simulink model "Simple_Model_Packaging_zhentouzhenwei3"  (R2022b)
settings: Solver=VariableStepAuto  StartTime=0.0  StopTime=0.05  RelTol=1e-3
InitFcn:
  | Parameter_Initialize_zhentouzhenwei
undefined symbols (not defined in the file or in its folder): gcbh, magnitude, model, rcfiltgaincompat
libraries: simulink x2, commrandsrc3 x2, commfilt2 x1, commchan3 x1, dspsigops x1, commdigbbndcpm2 x1, commseqgen3 x1, commutil2 x1, dsparch4 x1
settings Model: Creator=z0y  LastModifiedBy=z0y

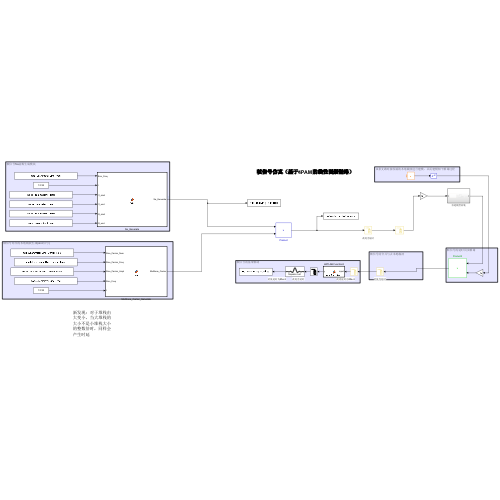
[thumbnail: Simulink's stored preview of the top-level diagram]
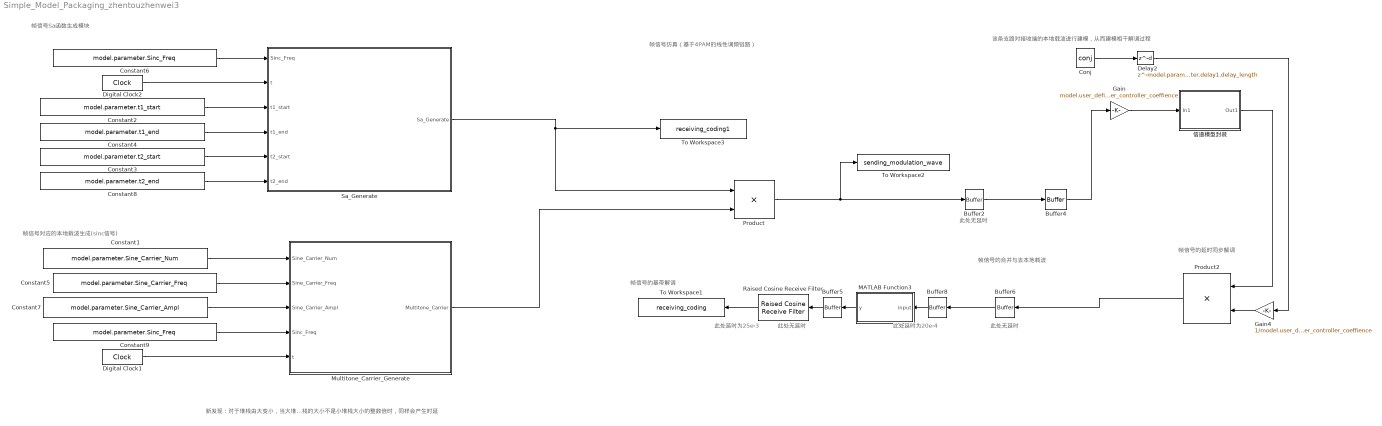
== system Simple_Model_Packaging_zhentouzhenwei3 ==
  note: 此处无延时
  note: 帧信号的延时同步解调
  note: 帧信号Sa函数生成模块
  note: 此处无延时
  note: 此处延时为25e-3
  note: 帧信号的基带解调
  note: 该条支路对接收端的本地载波进行建模，从而建模相干解调过程
  note: 帧信号的合并与去本地载波
  note: 帧信号仿真（基于4PAM的线性调频链路）
  note: 新发现：对于堆栈由大变小，当大堆栈的大小不是小堆栈大小的整数倍时，同样会产生时延
  note: 此处延时为20e-4
  note: 此处无延时
  note: 帧信号对应的本地载波生成(sinc信号)
  Buffer2 : Buffer  N=model.parameter.Buffer2.Output_buffer_size  OutputFrames=off
  Buffer4 : Buffer  N=model.parameter.Buffer4.Output_buffer_size  OutputFrames=off
  Buffer5 : Buffer  N=model.parameter.Buffer5.Output_buffer_size  OutputFrames=off
  Buffer6 : Buffer  N=model.parameter.Buffer6.Output_buffer_size  OutputFrames=off
  Buffer8 : Buffer  N=model.parameter.Buffer8.Output_buffer_size  OutputFrames=off
  Conj : Math  Operator=conj
  Constant1 : Constant  Value=model.parameter.Sine_Carrier_Num
  Constant2 : Constant  Value=model.parameter.t1_start
  Constant3 : Constant  Value=model.parameter.t2_start
  Constant4 : Constant  Value=model.parameter.t1_end
  Constant5 : Constant  Value=model.parameter.Sine_Carrier_Freq
  Constant6 : Constant  Value=model.parameter.Sinc_Freq
  Constant7 : Constant  Value=model.parameter.Sine_Carrier_Ampl
  Constant8 : Constant  Value=model.parameter.t2_end
  Constant9 : Constant  Value=model.parameter.Sinc_Freq
  Delay2 : Delay  DelayLength=model.parameter.delay1.delay_length  InitialCondition=0  InputProcessing=Columns as channels (frame based)
  Digital Clock1 : DigitalClock  SampleTime=model.parameter.Digital_Clock2.CarrierTs
  Digital Clock2 : DigitalClock  SampleTime=model.parameter.Digital_Clock2.CarrierTs
  Gain : Gain  Gain=model.user_defined.TR.Sig_power_controller_coeffience
  Gain4 : Gain  Gain=1/model.user_defined.TR.Sig_power_controller_coeffience
  MATLAB Function3 : MATLAB Function  TreatAsAtomicUnit=on
  Multitone_Carrier_Generate : MATLAB Function  TreatAsAtomicUnit=on
  Product : Product
  Product2 : Product
  Raised Cosine Receive Filter : commfilt2/Raised Cosine Receive Filter  filtType=Square root  R=model.parameter.Raised_Cosine_Receive_Filter.Rolloff_factor  filtSpan=model.parameter.Raised_Cosine_Receive_Filter.Filter_span_in_symbols  N=model.parameter.Raised_Cosine_Receive_Filter.Input_samples_per_symbol  downFactor=model.parameter.Raised_Cosine_Receive_Filter.Decimation_factor  downOffset=0  filterGain=rcfiltgaincompat(gcbh)  InputProcessing=Columns as channels (frame based)  RateOptions=Enforce single-rate processing  framing=Mute  checkCoeff=off  variableName=rcRxFilt  currentFiltSpan=10  D=5  inputOffset=0  sampMode=Mute  saveAsFlag=0  rateMode=Downsampling  checkGain=Normalized  launchFVT=on  roundingMode=Floor  overflowMode=off  coeffDataTypeStr=Inherit: Same word length as input  coeffMin=[]  coeffMax=[]  coeffLastDataTypeStr=Inherit: Same word length as input  accumDataTypeStr=Inherit: Same as product output  accumLastDataTypeStr=Inherit: Same as product output  outputDataTypeStr=Inherit: Same as accumulator  outputMin=[]  outputMax=[]  outputLastDataTypeStr=Inherit: Same as accumulator
  Sa_Generate : MATLAB Function  TreatAsAtomicUnit=on
  To Workspace1 : ToWorkspace  VariableName=receiving_coding  SaveFormat=Timeseries  SampleTime=-1
  To Workspace2 : ToWorkspace  VariableName=sending_modulation_wave  SaveFormat=Timeseries  SampleTime=-1
  To Workspace3 : ToWorkspace  VariableName=receiving_coding1  SaveFormat=Timeseries  SampleTime=-1
  信道模型封装 : Subsystem
  wires:
  Conj/1 -> Delay2/1
  Buffer8/1 -> MATLAB Function3/1(input)
  Gain/1 -> 信道模型封装/1(In1)
  Buffer4/1 -> Gain/1
  Delay2/1 -> Gain4/1
  Gain4/1 -> Product2/2
  MATLAB Function3/1(y) -> Buffer5/1
  信道模型封装/1(Out1) -> Product2/1
  Buffer5/1 -> Raised Cosine Receive Filter/1
  Buffer6/1 -> Buffer8/1
  Digital Clock1/1 -> Multitone_Carrier_Generate/5(t)
  Constant5/1 -> Multitone_Carrier_Generate/2(Sine_Carrier_Freq)
  Constant1/1 -> Multitone_Carrier_Generate/1(Sine_Carrier_Num)
  Constant7/1 -> Multitone_Carrier_Generate/3(Sine_Carrier_Ampl)
  Product/1 -> To Workspace2/1, Buffer2/1
  Product2/1 -> Buffer6/1
  Constant6/1 -> Sa_Generate/1(Sinc_Freq)
  Digital Clock2/1 -> Sa_Generate/2(t)
  Constant2/1 -> Sa_Generate/3(t1_start)
  Constant4/1 -> Sa_Generate/4(t1_end)
  Constant3/1 -> Sa_Generate/5(t2_start)
  Constant8/1 -> Sa_Generate/6(t2_end)
  Multitone_Carrier_Generate/1(Multitone_Carrier) -> Product/2
  Sa_Generate/1(Sa_Generate) -> Product/1, To Workspace3/1
  Raised Cosine Receive Filter/1 -> To Workspace1/1
  Buffer2/1 -> Buffer4/1
  Constant9/1 -> Multitone_Carrier_Generate/4(Sinc_Freq)

== system Simple_Model_Packaging_zhentouzhenwei3/信道模型封装 ==
  In1 : Inport
  AWGN Channel : commchan3/AWGN Channel  InputProcessing=Columns as channels (frame based)  seed=67  noiseMode="Signal to noise ratio  (SNR)"  EbNodB=10  EsNodB=10  SNRdB=model.parameter.Awgn.SNR  bitsPerSym=1  Ps=model.parameter.Awgn.input_power  Tsym=1  variance=1
  Add : Sum
  Buffer : Buffer  N=model.parameter.Buffer1.Output_buffer_size  OutputFrames=off
  NosieGen : Subsystem
  Out1 : Outport
  wires:
  AWGN Channel/1 -> Out1/1
  Add/1 -> AWGN Channel/1
  NosieGen/1(Jamming_Signal_Output) -> Buffer/1
  Buffer/1 -> Add/1  "TRSignal"
  In1/1 -> Add/2

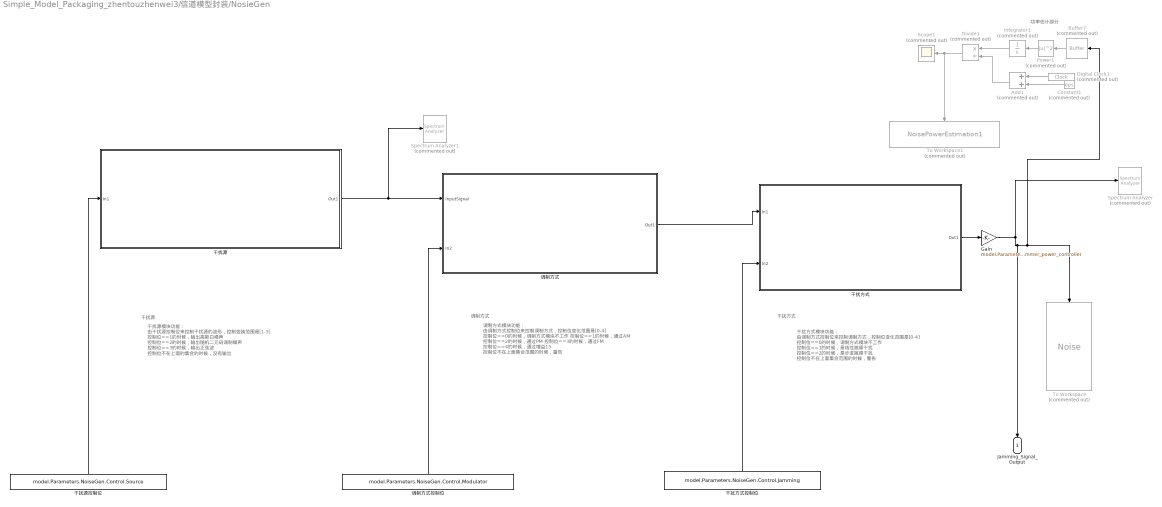
== system Simple_Model_Packaging_zhentouzhenwei3/信道模型封装/NosieGen ==
  note: 干扰源
  note: 调制方式
  note: 调制方式模块功能：
      | 由调制方式控制位来控制调制方式，控制位变化范围是[0-4]
      | 控制位==0的时候，调制方式模块不工作
      | 控制位==1的时候，通过AM
      | 控制位==2的时候，通过PM
      | 控制位==3的时候，通过FM
      | 控制位==4的时候，通过增益15
      | 控制位不在上面集合范围的时候，警告
  note: 干扰方式模块功能：
      | 由调制方式控制位来控制调制方式，控制位变化范围是[0-4]
      | 控制位==0的时候，调制方式模块不工作
      | 控制位==1的时候，是线性跳频干扰
      | 控制位==2的时候，是步进跳频干扰
      | 控制位不在上面集合范围的时候，警告
  note: 干扰源模块功能：
      | 由干扰源控制位来控制干扰源的波形，控制变换范围是[1-3]
      | 控制位==1的时候，输出高斯白噪声
      | 控制位==2的时候，输出随机二元码调制噪声
      | 控制位==3的时候，输出正弦波
      | 控制位不在上面的集合的时候，没有输出
  note: 干扰方式
  note: 功率估计部分
  Add1 : Sum  Commented=on
  Buffer7 : Buffer  Commented=on  N=1  OutputFrames=off
  Constant1 : Constant  Commented=on  Value=eps  SampleTime=model.Parameters.NoiseGen.NoiseTs
  Digital Clock1 : DigitalClock  Commented=on  SampleTime=model.Parameters.NoiseGen.NoiseTs
  Divide1 : Product  Commented=on  Inputs=*/
  Gain : Gain  Gain=model.Parameters.jammer_power_controller
  Integrator1 : Integrator  Commented=on
  Power1 : Math  Commented=on  Operator=magnitude^2
  Scope1 : Scope  Commented=on
  Spectrum Analyzer : SpectrumAnalyzer  Commented=on
  Spectrum Analyzer1 : SpectrumAnalyzer  Commented=on
  To Workspace : ToWorkspace  Commented=on  VariableName=Noise  SaveFormat=Timeseries  SampleTime=-1
  To Workspace1 : ToWorkspace  Commented=on  VariableName=NoisePowerEstimation1  SaveFormat=Timeseries  SampleTime=-1
  干扰方式 : Subsystem
  干扰方式控制位 : Constant  Value=model.Parameters.NoiseGen.Control.Jamming  SampleTime=Inf
  干扰源 : Subsystem
  干扰源控制位 : Constant  Value=model.Parameters.NoiseGen.Control.Source  SampleTime=Inf
  调制方式 : Subsystem
  调制方式控制位 : Constant  Value=model.Parameters.NoiseGen.Control.Modulator  SampleTime=Inf
  Jamming_Signal_Output : Outport
  wires:
  Digital Clock1/1 -> Add1/1
  Add1/1 -> Divide1/2
  干扰源控制位/1 -> 干扰源/1(In1)
  Power1/1 -> Integrator1/1
  Gain/1 -> Jamming_Signal_Output/1, Buffer7/1, To Workspace/1, Spectrum Analyzer/1
  Buffer7/1 -> Power1/1
  Divide1/1 -> Scope1/1, To Workspace1/1
  调制方式/1(Out1) -> 干扰方式/1(In1)
  Constant1/1 -> Add1/2
  调制方式控制位/1 -> 调制方式/2(In2)
  干扰源/1(Out1) -> Spectrum Analyzer1/1, 调制方式/1(InputSignal)
  干扰方式控制位/1 -> 干扰方式/2(In2)
  干扰方式/1(Out1) -> Gain/1
  Integrator1/1 -> Divide1/1

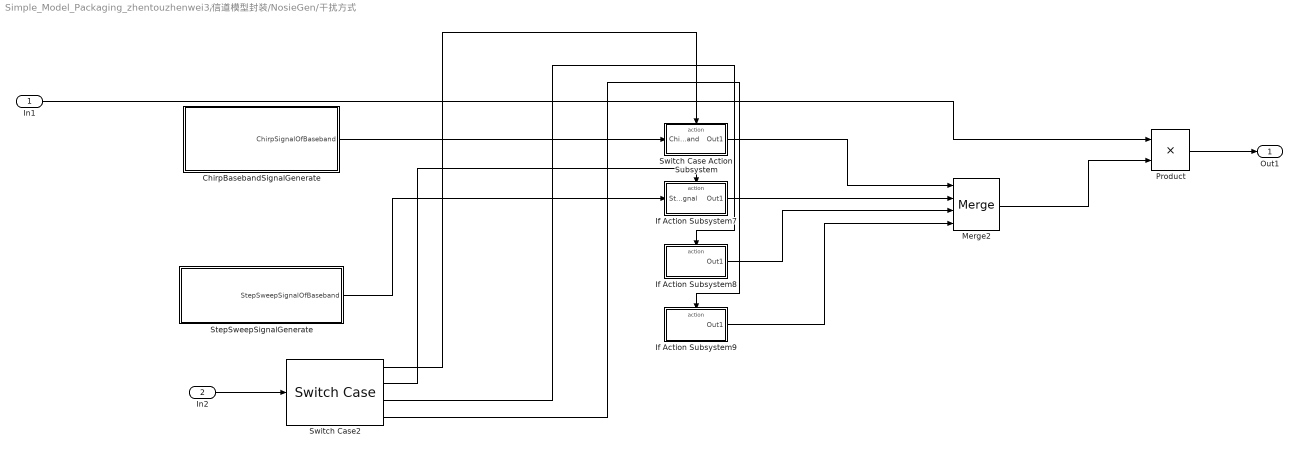
== system Simple_Model_Packaging_zhentouzhenwei3/信道模型封装/NosieGen/干扰方式 ==
  In1 : Inport
  In2 : Inport  Port=2
  ChirpBasebandSignalGenerate : Subsystem
      settings: AttributesFormatString=|
      | 线性调频模块：线性调频公式(y=exp(2*pi*(f_min*t+0.5*k_chirp*t^2)))
      | 输入参数：
      | 1. f_min,为线性调频信号的起始频率
      | 2.f_max为线性调频信号的终止频率
      | 3.T_chirp为线性调频信号的调频时间
      | 斜率k_sweep = (f_min-f_max)/T_chirp
  If Action Subsystem7 : Subsystem  TreatAsAtomicUnit=on
  If Action Subsystem8 : Subsystem  TreatAsAtomicUnit=on
  If Action Subsystem9 : Subsystem  TreatAsAtomicUnit=on
  Merge2 : Merge  Inputs=4
  Product : Product
  StepSweepSignalGenerate : Subsystem
  Switch Case Action Subsystem : Subsystem  TreatAsAtomicUnit=on
  Switch Case2 : SwitchCase  CaseConditions={1,2,3}
  Out1 : Outport
  wires:
  If Action Subsystem9/1(Out1) -> Merge2/4
  Switch Case Action Subsystem/1(Out1) -> Merge2/1
  If Action Subsystem8/1(Out1) -> Merge2/3
  Switch Case2/3 -> If Action Subsystem8/Action
  Switch Case2/1 -> Switch Case Action Subsystem/Action
  Switch Case2/2 -> If Action Subsystem7/Action
  Switch Case2/4 -> If Action Subsystem9/Action
  ChirpBasebandSignalGenerate/1(ChirpSignalOfBaseband) -> Switch Case Action Subsystem/1(ChirpSignalOfBaseband)
  If Action Subsystem7/1(Out1) -> Merge2/2
  Merge2/1 -> Product/2
  Product/1 -> Out1/1
  In1/1 -> Product/1
  In2/1 -> Switch Case2/1
  StepSweepSignalGenerate/1(StepSweepSignalOfBaseband) -> If Action Subsystem7/1(StepSweepSignal)

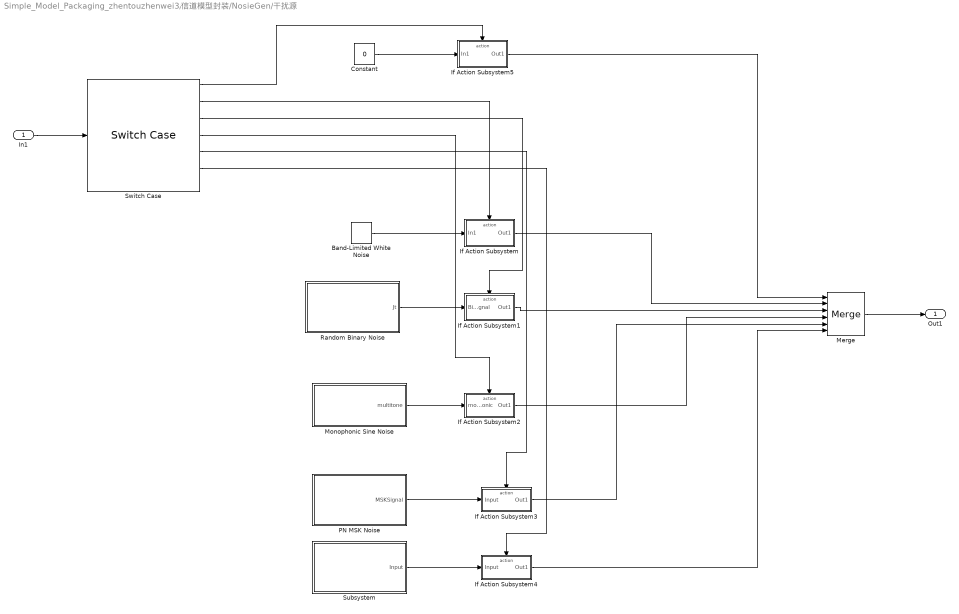
== system Simple_Model_Packaging_zhentouzhenwei3/信道模型封装/NosieGen/干扰源 ==
  In1 : Inport
  Band-Limited White Noise : simulink/Sources/Band-Limited White Noise  Cov=model.Parameters.NoiseGen.GaussPower  Ts=model.Parameters.NoiseGen.NoiseTs  seed=model.Parameters.NoiseGen.GaussSeed
  Constant : Constant  Value=0  SampleTime=model.Parameters.NoiseGen.NoiseTs
  If Action Subsystem : Subsystem  TreatAsAtomicUnit=on
  If Action Subsystem1 : Subsystem  TreatAsAtomicUnit=on
  If Action Subsystem2 : Subsystem  TreatAsAtomicUnit=on
  If Action Subsystem3 : Subsystem  TreatAsAtomicUnit=on
  If Action Subsystem4 : Subsystem  TreatAsAtomicUnit=on
  If Action Subsystem5 : Subsystem  TreatAsAtomicUnit=on
  Merge : Merge  Inputs=6
  Monophonic Sine Noise : Subsystem
  PN MSK Noise : Subsystem
  Random Binary Noise : Subsystem
  Subsystem : Subsystem
  Switch Case : SwitchCase  CaseConditions={0,1,2,3,4,5}
  Out1 : Outport
  wires:
  Switch Case/3 -> If Action Subsystem1/Action
  If Action Subsystem2/1(Out1) -> Merge/4
  Band-Limited White Noise/1 -> If Action Subsystem/1(In1)
  If Action Subsystem1/1(Out1) -> Merge/3
  Random Binary Noise/1(Jt) -> If Action Subsystem1/1(Binary_Random_Signal)
  Switch Case/4 -> If Action Subsystem2/Action
  Switch Case/2 -> If Action Subsystem/Action
  Merge/1 -> Out1/1
  In1/1 -> Switch Case/1
  Monophonic Sine Noise/1(multitone) -> If Action Subsystem2/1(monophonic)
  Switch Case/5 -> If Action Subsystem3/Action
  If Action Subsystem3/1(Out1) -> Merge/5
  If Action Subsystem/1(Out1) -> Merge/2
  PN MSK Noise/1(MSKSignal) -> If Action Subsystem3/1(Input)
  Switch Case/6 -> If Action Subsystem4/Action
  Subsystem/1(Input) -> If Action Subsystem4/1(Input)
  If Action Subsystem4/1(Out1) -> Merge/6
  Switch Case/1 -> If Action Subsystem5/Action
  Constant/1 -> If Action Subsystem5/1(In1)
  If Action Subsystem5/1(Out1) -> Merge/1

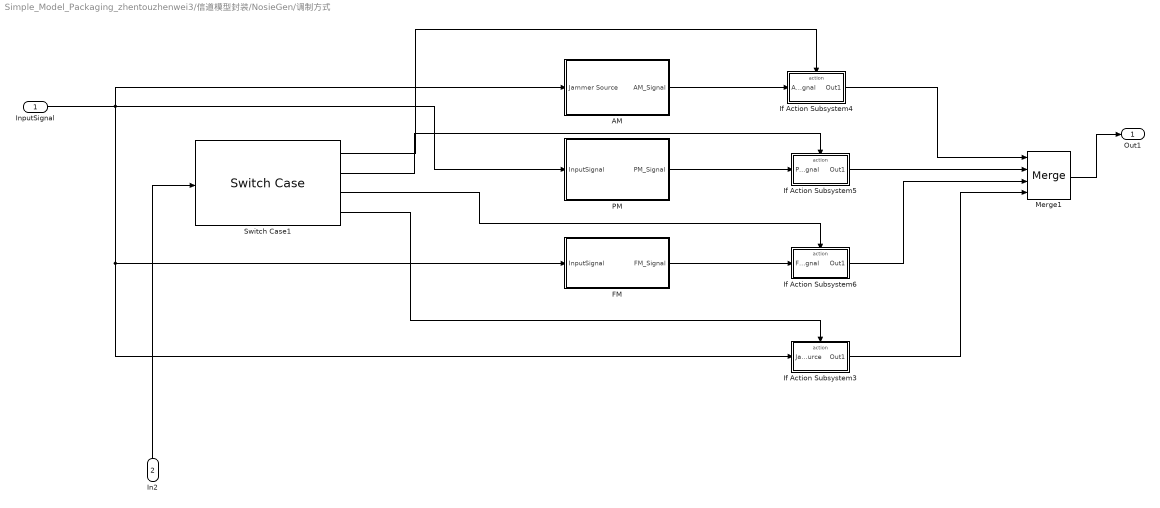
== system Simple_Model_Packaging_zhentouzhenwei3/信道模型封装/NosieGen/调制方式 ==
  InputSignal : Inport
  In2 : Inport  Port=2
  AM : Subsystem
  FM : Subsystem
  If Action Subsystem3 : Subsystem  TreatAsAtomicUnit=on
  If Action Subsystem4 : Subsystem  TreatAsAtomicUnit=on
  If Action Subsystem5 : Subsystem  TreatAsAtomicUnit=on
  If Action Subsystem6 : Subsystem  TreatAsAtomicUnit=on
  Merge1 : Merge  Inputs=4
  PM : Subsystem
  Switch Case1 : SwitchCase  CaseConditions={1,2,3}
  Out1 : Outport
  wires:
  In2/1 -> Switch Case1/1
  PM/1(PM_Signal) -> If Action Subsystem5/1(PM_Signal)
  Merge1/1 -> Out1/1
  If Action Subsystem3/1(Out1) -> Merge1/4
  If Action Subsystem6/1(Out1) -> Merge1/3
  If Action Subsystem5/1(Out1) -> Merge1/2
  InputSignal/1 -> FM/1(InputSignal), If Action Subsystem3/1(Jammer Source), PM/1(InputSignal), AM/1(Jammer Source)
  AM/1(AM_Signal) -> If Action Subsystem4/1(AM_Signal)
  Switch Case1/2 -> If Action Subsystem5/Action
  Switch Case1/3 -> If Action Subsystem6/Action
  Switch Case1/1 -> If Action Subsystem4/Action
  If Action Subsystem4/1(Out1) -> Merge1/1
  FM/1(FM_Signal) -> If Action Subsystem6/1(FM_Signal)
  Switch Case1/4 -> If Action Subsystem3/Action

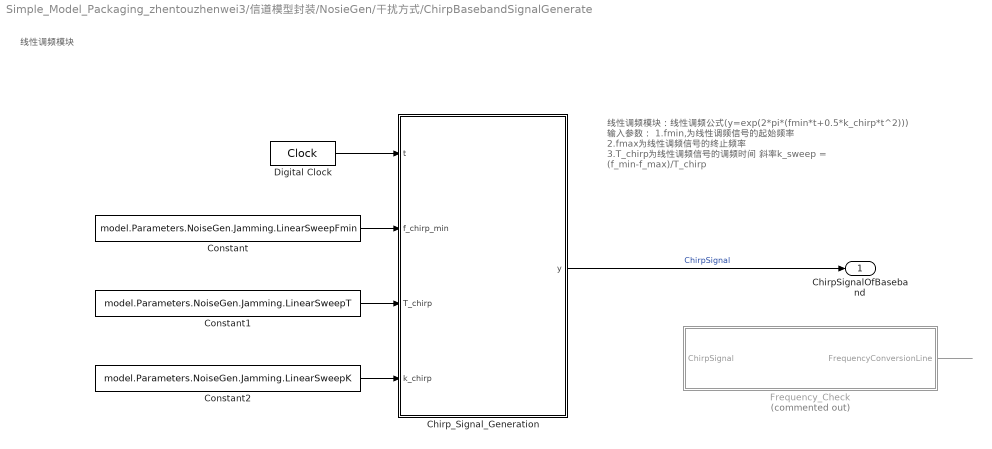
== system Simple_Model_Packaging_zhentouzhenwei3/信道模型封装/NosieGen/干扰方式/ChirpBasebandSignalGenerate ==
  note: 线性调频模块：线性调频公式(y=exp(2*pi*(fmin*t+0.5*k_chirp*t^2)))
      | 输入参数：
      | 1.fmin,为线性调频信号的起始频率
      | 2.fmax为线性调频信号的终止频率
      | 3.T_chirp为线性调频信号的调频时间
      | 斜率k_sweep = (f_min-f_max)/T_chirp
  note: 线性调频模块
  Chirp_Signal_Generation : MATLAB Function  TreatAsAtomicUnit=on
  Constant : Constant  Value=model.Parameters.NoiseGen.Jamming.LinearSweepFmin
  Constant1 : Constant  Value=model.Parameters.NoiseGen.Jamming.LinearSweepT
  Constant2 : Constant  Value=model.Parameters.NoiseGen.Jamming.LinearSweepK
  Digital Clock : DigitalClock  SampleTime=model.Parameters.NoiseGen.NoiseTs
  Frequency_Check : Subsystem  Commented=on
  ChirpSignalOfBaseband : Outport
  wires:
  Digital Clock/1 -> Chirp_Signal_Generation/1(t)
  Chirp_Signal_Generation/1(y) -> ChirpSignalOfBaseband/1  "ChirpSignal"
  Frequency_Check/1(FrequencyConversionLine) -> ?
  Constant/1 -> Chirp_Signal_Generation/2(f_chirp_min)
  Constant2/1 -> Chirp_Signal_Generation/4(k_chirp)
  Constant1/1 -> Chirp_Signal_Generation/3(T_chirp)

== system Simple_Model_Packaging_zhentouzhenwei3/信道模型封装/NosieGen/干扰方式/If Action Subsystem7 ==
  StepSweepSignal : Inport
  Action Port : ActionPort  ActionPortLabel=case [ 2 ]:
  Out1 : Outport
  wires:
  StepSweepSignal/1 -> Out1/1

== system Simple_Model_Packaging_zhentouzhenwei3/信道模型封装/NosieGen/干扰方式/If Action Subsystem8 ==
  Action Port : ActionPort  ActionPortLabel=case [ 3 ]:
  Constant : Constant  Value=10
  Constant1 : Constant  Value=0
  Real-Imag to Complex : RealImagToComplex
  Out1 : Outport
  wires:
  Constant/1 -> Real-Imag to Complex/1
  Real-Imag to Complex/1 -> Out1/1
  Constant1/1 -> Real-Imag to Complex/2

== system Simple_Model_Packaging_zhentouzhenwei3/信道模型封装/NosieGen/干扰方式/If Action Subsystem9 ==
  Action Port : ActionPort  ActionPortLabel=default:
  Constant : Constant
  Constant1 : Constant  Value=0
  Real-Imag to Complex : RealImagToComplex
  Out1 : Outport
  wires:
  Constant/1 -> Real-Imag to Complex/1
  Real-Imag to Complex/1 -> Out1/1
  Constant1/1 -> Real-Imag to Complex/2

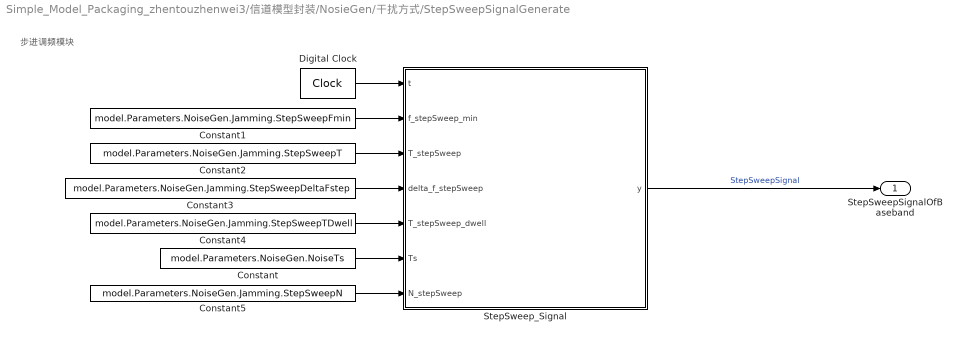
== system Simple_Model_Packaging_zhentouzhenwei3/信道模型封装/NosieGen/干扰方式/StepSweepSignalGenerate ==
  note: 步进调频模块
  Constant : Constant  Value=model.Parameters.NoiseGen.NoiseTs
  Constant1 : Constant  Value=model.Parameters.NoiseGen.Jamming.StepSweepFmin
  Constant2 : Constant  Value=model.Parameters.NoiseGen.Jamming.StepSweepT
  Constant3 : Constant  Value=model.Parameters.NoiseGen.Jamming.StepSweepDeltaFstep
  Constant4 : Constant  Value=model.Parameters.NoiseGen.Jamming.StepSweepTDwell
  Constant5 : Constant  Value=model.Parameters.NoiseGen.Jamming.StepSweepN
  Digital Clock : DigitalClock  SampleTime=model.Parameters.NoiseGen.NoiseTs
  StepSweep_Signal : MATLAB Function  TreatAsAtomicUnit=on
  StepSweepSignalOfBaseband : Outport
  wires:
  Digital Clock/1 -> StepSweep_Signal/1(t)
  StepSweep_Signal/1(y) -> StepSweepSignalOfBaseband/1  "StepSweepSignal"
  Constant/1 -> StepSweep_Signal/6(Ts)
  Constant1/1 -> StepSweep_Signal/2(f_stepSweep_min)
  Constant2/1 -> StepSweep_Signal/3(T_stepSweep)
  Constant3/1 -> StepSweep_Signal/4(delta_f_stepSweep)
  Constant4/1 -> StepSweep_Signal/5(T_stepSweep_dwell)
  Constant5/1 -> StepSweep_Signal/7(N_stepSweep)

== system Simple_Model_Packaging_zhentouzhenwei3/信道模型封装/NosieGen/干扰方式/Switch Case Action Subsystem ==
  ChirpSignalOfBaseband : Inport
  Action Port : ActionPort  ActionPortLabel=case [ 1 ]:
  Out1 : Outport
  wires:
  ChirpSignalOfBaseband/1 -> Out1/1

== system Simple_Model_Packaging_zhentouzhenwei3/信道模型封装/NosieGen/干扰源/If Action Subsystem ==
  In1 : Inport
  Action Port : ActionPort  ActionPortLabel=case [ 1 ]:
  Out1 : Outport
  wires:
  In1/1 -> Out1/1

== system Simple_Model_Packaging_zhentouzhenwei3/信道模型封装/NosieGen/干扰源/If Action Subsystem1 ==
  Binary_Random_Signal : Inport
  Action Port : ActionPort  ActionPortLabel=case [ 2 ]:
  Out1 : Outport
  wires:
  Binary_Random_Signal/1 -> Out1/1

== system Simple_Model_Packaging_zhentouzhenwei3/信道模型封装/NosieGen/干扰源/If Action Subsystem2 ==
  monophonic : Inport
  Action Port : ActionPort  ActionPortLabel=case [ 3 ]:
  Out1 : Outport
  wires:
  monophonic/1 -> Out1/1

== system Simple_Model_Packaging_zhentouzhenwei3/信道模型封装/NosieGen/干扰源/If Action Subsystem3 ==
  Input : Inport
  Action Port : ActionPort  ActionPortLabel=case [ 4 ]:
  Out1 : Outport
  wires:
  Input/1 -> Out1/1

== system Simple_Model_Packaging_zhentouzhenwei3/信道模型封装/NosieGen/干扰源/If Action Subsystem4 ==
  Input : Inport
  Action Port : ActionPort  ActionPortLabel=case [ 5 ]:
  Out1 : Outport
  wires:
  Input/1 -> Out1/1

== system Simple_Model_Packaging_zhentouzhenwei3/信道模型封装/NosieGen/干扰源/If Action Subsystem5 ==
  In1 : Inport
  Action Port : ActionPort  ActionPortLabel=case [ 0 ]:
  Out1 : Outport
  wires:
  In1/1 -> Out1/1

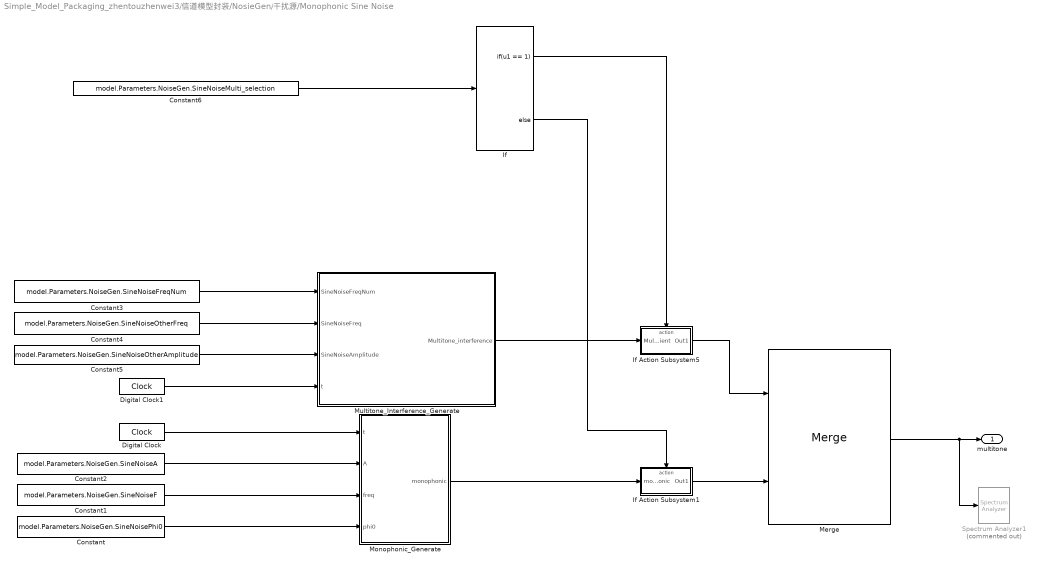
== system Simple_Model_Packaging_zhentouzhenwei3/信道模型封装/NosieGen/干扰源/Monophonic Sine Noise ==
  Constant : Constant  Value=model.Parameters.NoiseGen.SineNoisePhi0
  Constant1 : Constant  Value=model.Parameters.NoiseGen.SineNoiseF
  Constant2 : Constant  Value=model.Parameters.NoiseGen.SineNoiseA
  Constant3 : Constant  Value=model.Parameters.NoiseGen.SineNoiseFreqNum
  Constant4 : Constant  Value=model.Parameters.NoiseGen.SineNoiseOtherFreq
  Constant5 : Constant  Value=model.Parameters.NoiseGen.SineNoiseOtherAmplitude
  Constant6 : Constant  Value=model.Parameters.NoiseGen.SineNoiseMulti_selection
  Digital Clock : DigitalClock  SampleTime=model.Parameters.NoiseGen.NoiseTs
  Digital Clock1 : DigitalClock  SampleTime=model.Parameters.NoiseGen.NoiseTs
  If : If  IfExpression=u1 == 1
  If Action Subsystem1 : Subsystem  TreatAsAtomicUnit=on
  If Action Subsystem5 : Subsystem  TreatAsAtomicUnit=on
  Merge : Merge
  Monophonic_Generate : MATLAB Function  TreatAsAtomicUnit=on
  Multitone_Interference_Generate : MATLAB Function  TreatAsAtomicUnit=on
  Spectrum Analyzer1 : SpectrumAnalyzer  Commented=on
  multitone : Outport
  wires:
  Digital Clock/1 -> Monophonic_Generate/1(t)
  Constant/1 -> Monophonic_Generate/4(phi0)
  Constant2/1 -> Monophonic_Generate/2(A)
  Constant1/1 -> Monophonic_Generate/3(freq)
  Constant3/1 -> Multitone_Interference_Generate/1(SineNoiseFreqNum)
  Constant4/1 -> Multitone_Interference_Generate/2(SineNoiseFreq)
  Constant5/1 -> Multitone_Interference_Generate/3(SineNoiseAmplitude)
  Multitone_Interference_Generate/1(Multitone_interference) -> If Action Subsystem5/1(Multitone_multiplicative_coefficient)
  Merge/1 -> Spectrum Analyzer1/1, multitone/1
  Digital Clock1/1 -> Multitone_Interference_Generate/4(t)
  Constant6/1 -> If/1
  If/1 -> If Action Subsystem5/Action
  If/2 -> If Action Subsystem1/Action
  If Action Subsystem5/1(Out1) -> Merge/1
  Monophonic_Generate/1(monophonic) -> If Action Subsystem1/1(monophonic)
  If Action Subsystem1/1(Out1) -> Merge/2

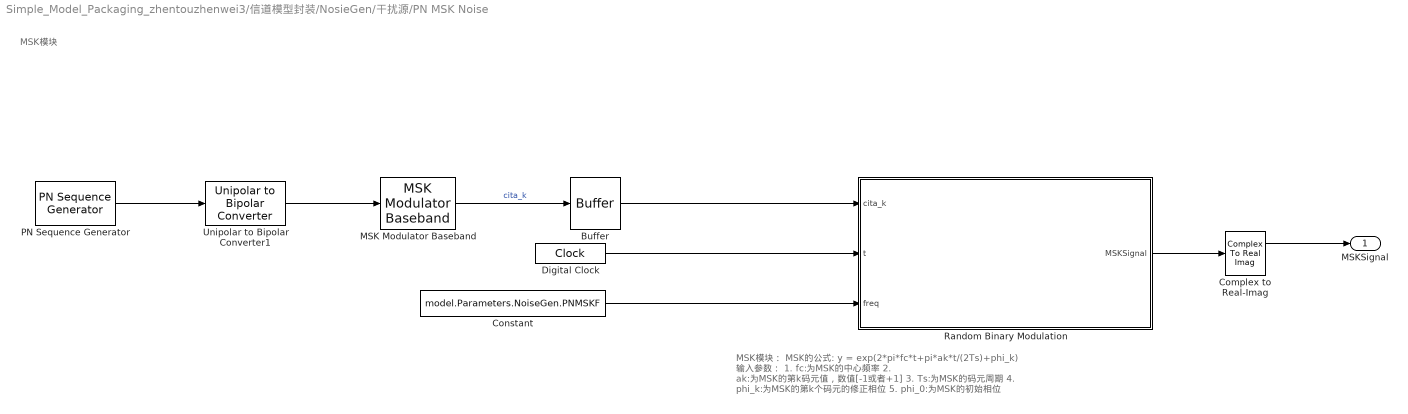
== system Simple_Model_Packaging_zhentouzhenwei3/信道模型封装/NosieGen/干扰源/PN MSK Noise ==
  note: MSK模块
  note: MSK模块：
      | MSK的公式: y = exp(2*pi*fc*t+pi*ak*t/(2Ts)+phi_k)
      | 输入参数：
      | 1. fc:为MSK的中心频率
      | 2. ak:为MSK的第k码元值，数值[-1或者+1]
      | 3. Ts:为MSK的码元周期
      | 4. phi_k:为MSK的第k个码元的修正相位
      | 5. phi_0:为MSK的初始相位
  Buffer : Buffer  N=1  OutputFrames=off
  Complex to Real-Imag : ComplexToRealImag
  Constant : Constant  Value=model.Parameters.NoiseGen.PNMSKF
  Digital Clock : DigitalClock  SampleTime=model.Parameters.NoiseGen.NoiseTs
  MSK Modulator Baseband : commdigbbndcpm2/MSK Modulator Baseband  inputType=Integer  phaseOffset=model.Parameters.NoiseGen.PNMSKPhi0  samplesPerSymbol=model.Parameters.NoiseGen.PNMSKM  RateOptions=Enforce single-rate processing  outDataType=double
  PN Sequence Generator : commseqgen3/PN Sequence Generator  poly=model.Parameters.NoiseGen.PNMSKPolynomial  ini_sta=model.Parameters.NoiseGen.PNMSKInitialstate  outBitMaskSource=Dialog parameter  shift=0  outVarSiz=off  maxOutSizeMode=Dialog parameter  maxOutSize=[10 1]  Ts=model.Parameters.NoiseGen.PNMSKM * model.Parameters.NoiseGen.NoiseTs  sampPerFrame=1  reset=off  bitPackedOutputs=off  outDataType=double  numPackedBits=8  bitPackDataSigned=off  bitPackedOutDType=double
      settings: LibrarySourceBlock=|
      | commhdlsource/PN Sequence
      | Generator
  Random Binary Modulation : MATLAB Function  TreatAsAtomicUnit=on
  Unipolar to Bipolar Converter1 : commutil2/Unipolar to Bipolar Converter  M=2  polarity=Positive  dataType=Inherit via internal rule
  MSKSignal : Outport  OutDataTypeStr=double
  wires:
  Digital Clock/1 -> Random Binary Modulation/2(t)
  Unipolar to Bipolar Converter1/1 -> MSK Modulator Baseband/1
  PN Sequence Generator/1 -> Unipolar to Bipolar Converter1/1
  Constant/1 -> Random Binary Modulation/3(freq)
  MSK Modulator Baseband/1 -> Buffer/1  "cita_k"
  Buffer/1 -> Random Binary Modulation/1(cita_k)
  Random Binary Modulation/1(MSKSignal) -> Complex to Real-Imag/1
  Complex to Real-Imag/1 -> MSKSignal/1

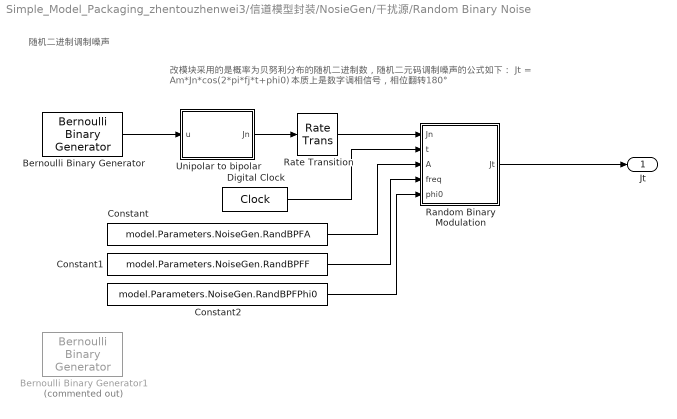
== system Simple_Model_Packaging_zhentouzhenwei3/信道模型封装/NosieGen/干扰源/Random Binary Noise ==
  note: 改模块采用的是概率为贝努利分布的随机二进制数，随机二元码调制噪声的公式如下：
      | Jt = Am*Jn*cos(2*pi*fj*t+phi0)
      | 本质上是数字调相信号，相位翻转180°
  note: 随机二进制调制噪声
  Bernoulli Binary Generator : commrandsrc3/Bernoulli Binary Generator  ProbabilityOfZero=model.Parameters.NoiseGen.RandBFZero  SeedSource=Auto  Seed=0  SampleTime=model.Parameters.NoiseGen.NoiseTs  SamplesPerFrame=1  OutputDataType=double  SimulateUsing=Interpreted execution
  Bernoulli Binary Generator1 : commrandsrc3/Bernoulli Binary Generator  Commented=on  ProbabilityOfZero=model.Parameters.NoiseGen.RandBFZero  SeedSource=Auto  Seed=0  SampleTime=model.Parameters.NoiseGen.PRCodeTs  SamplesPerFrame=1  OutputDataType=double  SimulateUsing=Interpreted execution
  Constant : Constant  Value=model.Parameters.NoiseGen.RandBPFA
  Constant1 : Constant  Value=model.Parameters.NoiseGen.RandBPFF
  Constant2 : Constant  Value=model.Parameters.NoiseGen.RandBPFPhi0
  Digital Clock : DigitalClock  SampleTime=model.Parameters.NoiseGen.NoiseTs
  Random Binary Modulation : MATLAB Function  TreatAsAtomicUnit=on
  Rate Transition : RateTransition
  Unipolar to bipolar : MATLAB Function  TreatAsAtomicUnit=on
  Jt : Outport
  wires:
  Unipolar to bipolar/1(Jn) -> Rate Transition/1
  Bernoulli Binary Generator/1 -> Unipolar to bipolar/1(u)
  Random Binary Modulation/1(Jt) -> Jt/1
  Digital Clock/1 -> Random Binary Modulation/2(t)
  Constant/1 -> Random Binary Modulation/3(A)
  Constant1/1 -> Random Binary Modulation/4(freq)
  Constant2/1 -> Random Binary Modulation/5(phi0)
  Rate Transition/1 -> Random Binary Modulation/1(Jn)

== system Simple_Model_Packaging_zhentouzhenwei3/信道模型封装/NosieGen/干扰源/Subsystem ==
  Band-Limited White Noise : simulink/Sources/Band-Limited White Noise  Cov=model.Parameters.NoiseGen.RFNoisePower  Ts=model.Parameters.NoiseGen.NoiseTs  seed=model.Parameters.NoiseGen.RFNoiseSeed
  Filter : dsparch4/Biquad Filter  Tag=BlockMethodSubSystem  FilterSource=Filter object  CoeffSource=Specify via dialog  FilterObject=model.Parameters.NoiseGen.RFNoiseFilterObj  IIRFiltStruct=Direct form II  BiQuadCoeffs=[1 2 1 1 -1.48178412853867569 0.831585910854089061;1 2 1 1 -1.27721148327892942 0.578720214976092495;1 2 1 1 -1.14298050253990113 0.412801598096188771;1 2 1 1 -1.06189684687510177 0.31257668783031084;1 2 1 1 -1.02371666858405952 0.265383392069520774]  ScaleValues=[0.0874504455788533558;0.0753771829242907976;0.0674552738890718956;0.0626699602388022664;0.0604166808713653344;1]  IC=0  ICnum=0  ICden=0  a0Flag=Warning  optimizeScaleValues=on  ScaleValueMode=Specify via input port (g)  roundingMode=Floor  overflowMode=off  scaleValueFracLength=14  denProdOutputFracLength=30  denAccumFracLength=30  secondMemoryFracLength=15
  Input : Outport
  wires:
  Band-Limited White Noise/1 -> Filter/1
  Filter/1 -> Input/1

== system Simple_Model_Packaging_zhentouzhenwei3/信道模型封装/NosieGen/调制方式/AM ==
  Jammer Source : Inport
  AM_Carrier : MATLAB Function  TreatAsAtomicUnit=on
  Constant : Constant  Value=model.Parameters.NoiseGen.Modulator.AMA
  Constant1 : Constant  Value=model.Parameters.NoiseGen.Modulator.AMF
  Constant2 : Constant  Value=model.Parameters.NoiseGen.Modulator.Ma
  Digital Clock : DigitalClock  SampleTime=model.Parameters.NoiseGen.NoiseTs
  AM_Signal : Outport
  wires:
  Digital Clock/1 -> AM_Carrier/1(t)
  AM_Carrier/1(y) -> AM_Signal/1  "ChirpSignal"
  Constant2/1 -> AM_Carrier/5(Ma)
  Constant1/1 -> AM_Carrier/3(freq)
  Constant/1 -> AM_Carrier/2(A)
  Jammer Source/1 -> AM_Carrier/4(carrier_low_freq)

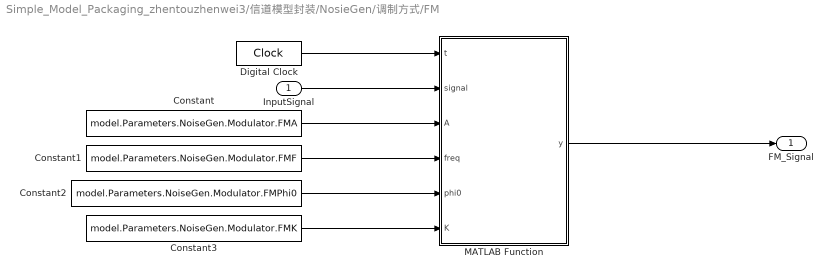
== system Simple_Model_Packaging_zhentouzhenwei3/信道模型封装/NosieGen/调制方式/FM ==
  InputSignal : Inport
  Constant : Constant  Value=model.Parameters.NoiseGen.Modulator.FMA
  Constant1 : Constant  Value=model.Parameters.NoiseGen.Modulator.FMF
  Constant2 : Constant  Value=model.Parameters.NoiseGen.Modulator.FMPhi0
  Constant3 : Constant  Value=model.Parameters.NoiseGen.Modulator.FMK
  Digital Clock : DigitalClock  SampleTime=model.Parameters.NoiseGen.NoiseTs
  MATLAB Function : MATLAB Function  TreatAsAtomicUnit=on
  FM_Signal : Outport
  wires:
  Digital Clock/1 -> MATLAB Function/1(t)
  MATLAB Function/1(y) -> FM_Signal/1
  InputSignal/1 -> MATLAB Function/2(signal)
  Constant/1 -> MATLAB Function/3(A)
  Constant1/1 -> MATLAB Function/4(freq)
  Constant2/1 -> MATLAB Function/5(phi0)
  Constant3/1 -> MATLAB Function/6(K)

== system Simple_Model_Packaging_zhentouzhenwei3/信道模型封装/NosieGen/调制方式/If Action Subsystem3 ==
  Jammer Source : Inport
  Action Port : ActionPort  ActionPortLabel=default:
  Out1 : Outport
  wires:
  Jammer Source/1 -> Out1/1

== system Simple_Model_Packaging_zhentouzhenwei3/信道模型封装/NosieGen/调制方式/If Action Subsystem4 ==
  AM_Signal : Inport
  Action Port : ActionPort  ActionPortLabel=case [ 1 ]:
  Out1 : Outport
  wires:
  AM_Signal/1 -> Out1/1

== system Simple_Model_Packaging_zhentouzhenwei3/信道模型封装/NosieGen/调制方式/If Action Subsystem5 ==
  PM_Signal : Inport
  Action Port : ActionPort  ActionPortLabel=case [ 2 ]:
  Out1 : Outport
  wires:
  PM_Signal/1 -> Out1/1

== system Simple_Model_Packaging_zhentouzhenwei3/信道模型封装/NosieGen/调制方式/If Action Subsystem6 ==
  FM_Signal : Inport
  Action Port : ActionPort  ActionPortLabel=case [ 3 ]:
  Out1 : Outport
  wires:
  FM_Signal/1 -> Out1/1

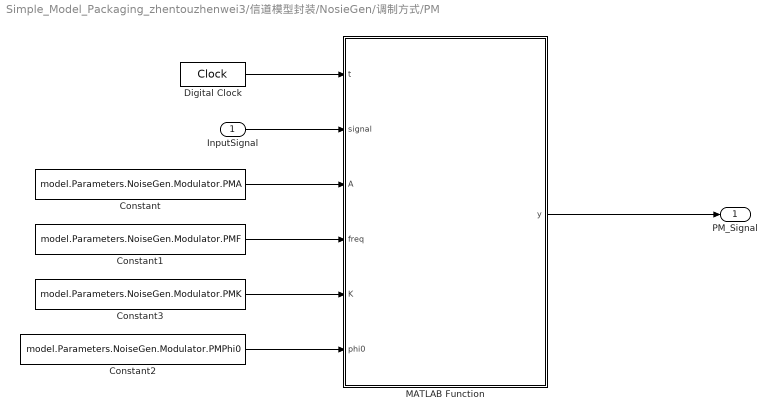
== system Simple_Model_Packaging_zhentouzhenwei3/信道模型封装/NosieGen/调制方式/PM ==
  InputSignal : Inport
  Constant : Constant  Value=model.Parameters.NoiseGen.Modulator.PMA
  Constant1 : Constant  Value=model.Parameters.NoiseGen.Modulator.PMF
  Constant2 : Constant  Value=model.Parameters.NoiseGen.Modulator.PMPhi0
  Constant3 : Constant  Value=model.Parameters.NoiseGen.Modulator.PMK
  Digital Clock : DigitalClock  SampleTime=model.Parameters.NoiseGen.NoiseTs
  MATLAB Function : MATLAB Function  TreatAsAtomicUnit=on
  PM_Signal : Outport
  wires:
  Digital Clock/1 -> MATLAB Function/1(t)
  InputSignal/1 -> MATLAB Function/2(signal)
  MATLAB Function/1(y) -> PM_Signal/1
  Constant/1 -> MATLAB Function/3(A)
  Constant1/1 -> MATLAB Function/4(freq)
  Constant3/1 -> MATLAB Function/5(K)
  Constant2/1 -> MATLAB Function/6(phi0)

== system Simple_Model_Packaging_zhentouzhenwei3/信道模型封装/NosieGen/干扰方式/ChirpBasebandSignalGenerate/Frequency_Check ==
  ChirpSignal : Inport
  Derivative : Derivative
  Phase Extractor : dspsigops/Phase Extractor  TreatFramesIndependently=off  SimulateUsing=Code generation
  FrequencyConversionLine : Outport
  wires:
  ChirpSignal/1 -> Phase Extractor/1
  Phase Extractor/1 -> Derivative/1
  Derivative/1 -> FrequencyConversionLine/1

== system Simple_Model_Packaging_zhentouzhenwei3/信道模型封装/NosieGen/干扰源/Monophonic Sine Noise/If Action Subsystem1 ==
  monophonic : Inport
  Action Port : ActionPort  ActionPortLabel=else
  Out1 : Outport
  wires:
  monophonic/1 -> Out1/1

== system Simple_Model_Packaging_zhentouzhenwei3/信道模型封装/NosieGen/干扰源/Monophonic Sine Noise/If Action Subsystem5 ==
  Multitone_multiplicative_coefficient : Inport
  Action Port : ActionPort  ActionPortLabel=if(u1 == 1)
  Out1 : Outport
  wires:
  Multitone_multiplicative_coefficient/1 -> Out1/1

== matlab function Simple_Model_Packaging_zhentouzhenwei3/信道模型封装/NosieGen/干扰源/Monophonic Sine Noise/Multitone_Interference_Generate ==
  data: SineNoiseFreqNum input; Multitone_interference output; SineNoiseFreq input; SineNoiseAmplitude input; t input
function Multitone_interference = fcn(SineNoiseFreqNum, SineNoiseFreq, SineNoiseAmplitude, t)
Multitone_interference = 0;

for index = 1:SineNoiseFreqNum
    Multitone_interference_subinterference = SineNoiseAmplitude(index) * sin(2*pi*SineNoiseFreq(index)*t);
    Multitone_interference = Multitone_interference + Multitone_interference_subinterference;
end

== matlab function Simple_Model_Packaging_zhentouzhenwei3/信道模型封装/NosieGen/调制方式/FM/MATLAB Function ==
  data: t input; signal input; y output; A input; freq input; phi0 input; K input
function y = FM(t, signal, A, freq, phi0, K)
   y = A*cos(2*pi*(freq+K*signal)*t+phi0) ;
end

== matlab function Simple_Model_Packaging_zhentouzhenwei3/信道模型封装/NosieGen/调制方式/PM/MATLAB Function ==
  data: t input; signal input; y output; A input; freq input; K input; phi0 input
function y = PM(t, signal, A, freq, K, phi0)
   y = A*cos(2*pi*freq*t+K*signal+phi0) ;
end

== matlab function Simple_Model_Packaging_zhentouzhenwei3/Multitone_Carrier_Generate ==
  data: Sine_Carrier_Num input; Multitone_Carrier output; Sine_Carrier_Freq input; Sine_Carrier_Ampl input; Sinc_Freq input; t input
function Multitone_Carrier = fcn(Sine_Carrier_Num, Sine_Carrier_Freq, Sine_Carrier_Ampl,Sinc_Freq, t)
    Multitone_Carrier = complex(0);
    Num_sidelobe = 9 ; % 定义最后生成信号的两个主瓣之间的旁瓣的个数
    T_between = (Num_sidelobe + 2)/Sinc_Freq; % 相邻两个重复单元间隔多久。这个也可以从最后生成信号的两个主峰间的时间间隔可以看出来
    t = mod(t,T_between);
    for index = 1:Sine_Carrier_Num
            Multitone_subCarrier = Sine_Carrier_Ampl(index) * exp(1j*2*pi*Sine_Carrier_Freq(index)*t);
            Multitone_Carrier = Multitone_Carrier + Multitone_subCarrier;
    end
end

== matlab function Simple_Model_Packaging_zhentouzhenwei3/Sa_Generate ==
  data: Sa_Generate output; Sinc_Freq input; t input; t1_start input; t1_end input; t2_start input; t2_end input
function Sa_Generate = fcn(Sinc_Freq, t,t1_start , t1_end,t2_start,t2_end)
    Num_sidelobe = 9 ; % 定义最后生成信号的两个主瓣之间的旁瓣的个数
    T_between = (Num_sidelobe + 2)/Sinc_Freq; % 相邻两个重复单元间隔多久。这个也可以从最后生成信号的两个主峰间的时间间隔可以看出来
    if ((t>=t1_start)&&(t<=t1_end))||((t>=t2_start)&&(t<=t2_end))
    t = mod(t,T_between);
    Sa_Generate = sinc(t*Sinc_Freq-5);
    else
        Sa_Generate = 0;
    end
end

== matlab function Simple_Model_Packaging_zhentouzhenwei3/信道模型封装/NosieGen/干扰方式/ChirpBasebandSignalGenerate/Chirp_Signal_Generation ==
  data: y output; t input; f_chirp_min input; T_chirp input; k_chirp input
function y = ChirpSignal(t, f_chirp_min, T_chirp, k_chirp)
    t = mod(t,T_chirp);
    y = exp(1i*2*pi*(f_chirp_min*t+0.5*k_chirp*t^2));
end

== matlab function Simple_Model_Packaging_zhentouzhenwei3/信道模型封装/NosieGen/干扰源/Monophonic Sine Noise/Monophonic_Generate ==
  data: t input; A input; freq input; monophonic output; phi0 input
function monophonic = MonophonicGenerate(t, A, freq, phi0)
    monophonic = A * sin(2*pi*freq*t+phi0);
end

== matlab function Simple_Model_Packaging_zhentouzhenwei3/信道模型封装/NosieGen/干扰源/Random Binary Noise/Random Binary Modulation ==
  data: Jn input; Jt output; t input; A input; freq input; phi0 input
function Jt = fcn(Jn,t,A,freq,phi0)
    Jt = A*Jn*cos(2*pi*freq*t+phi0);
end

== matlab function Simple_Model_Packaging_zhentouzhenwei3/MATLAB Function3 ==
  data: y output; input input
% function y = carrierGenerator(t)
%     fc = 5e6;
%     y = exp(1i*2*pi*fc*t);

function y = rateTransition(input)
    p = 1;
    q = 10;
    y = resample(input,p,q);
%     y(1:10) = repmat(y(10),1,10);
%     y(end-9:end) = repmat(y(end-9),1,10);
end

== matlab function Simple_Model_Packaging_zhentouzhenwei3/信道模型封装/NosieGen/干扰源/Random Binary Noise/Unipolar to bipolar ==
  data: u input; Jn output
function Jn= fcn(u)
    Jn = 2*u-1;
end

== matlab function Simple_Model_Packaging_zhentouzhenwei3/信道模型封装/NosieGen/干扰方式/StepSweepSignalGenerate/StepSweep_Signal ==
  data: y output; t input; f_stepSweep_min input; T_stepSweep input; delta_f_stepSweep input; T_stepSweep_dwell input; Ts input; N_stepSweep input
function y  = StepSweep(t, f_stepSweep_min, T_stepSweep, delta_f_stepSweep, T_stepSweep_dwell, Ts, N_stepSweep)
    a = mod(t,T_stepSweep)+Ts/10000;
    b = fix(a/T_stepSweep_dwell);
    if b == N_stepSweep
        b = N_stepSweep - 1;
    end
    f = (f_stepSweep_min + b*delta_f_stepSweep);
    y = exp(1i*2*pi*f*t);
end

== matlab function Simple_Model_Packaging_zhentouzhenwei3/信道模型封装/NosieGen/干扰源/PN MSK Noise/Random Binary Modulation ==
  data: cita_k input; MSKSignal output; t input; freq input
function MSKSignal = fcn(cita_k,t, freq)
    MSKSignal = cita_k * cos(2*pi*freq*t);
end

== matlab function Simple_Model_Packaging_zhentouzhenwei3/信道模型封装/NosieGen/调制方式/AM/AM_Carrier ==
  data: y output; t input; A input; freq input; carrier_low_freq input; Ma input
function y = AM_Carrier(t, A, freq, carrier_low_freq, Ma)
    y = A*(1+Ma*carrier_low_freq)*cos(2*pi*freq*t);
end
